simulink model "lab21"  (R2016a)
settings: Solver=VariableStepAuto  StartTime=0.0  StopTime=10.0  RelTol=1e-3
libraries: visionsources x2
settings Model: Creator=Auroshis  LastModifiedBy=Auroshis

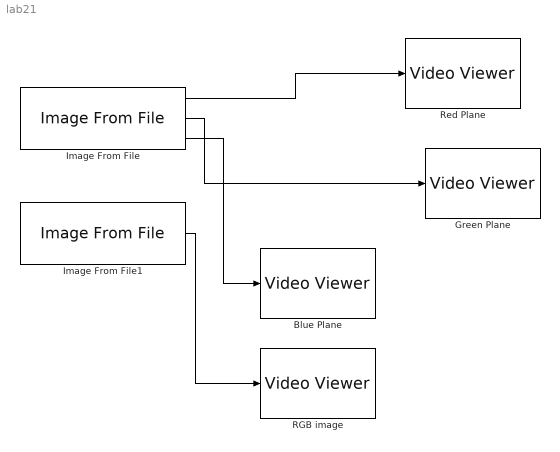
== system lab21 ==
  Blue Plane : VideoViewer  FigPos=[609.8 405.2 409.6 300]
  Green Plane : VideoViewer  FigPos=[606.6 802.8 409.6 300]
  Image From File : visionsources/Image From File  Tag=vipblks_nd  FileName=peppers.png  imagePorts=Separate color signals  Ts=0.1  ImageDataType=Inherit from input image  Signed=on  WordLength=16  sdImageDataType=uint(8)  FractionLengthMode=User-defined  FractionLength=15  OutPortLabels=R|G|B
  Image From File1 : visionsources/Image From File  Tag=vipblks_nd  FileName=peppers.png  imagePorts=One multidimensional signal  Ts=0.1  ImageDataType=Inherit from input image  Signed=on  WordLength=16  sdImageDataType=uint(8)  FractionLengthMode=User-defined  FractionLength=15  OutPortLabels=R|G|B
  "RGB image " : VideoViewer  FigPos=[197 411.6 409.6 300]
  Red Plane : VideoViewer  FigPos=[193.8 802 409.6 300]
  wires:
  Image From File/1 -> Red Plane/1
  Image From File/3 -> Blue Plane/1
  Image From File/2 -> Green Plane/1
  Image From File1/1 -> "RGB image "/1
